simulink model "CarHalf_Vertical"  (R2018b)
settings: Solver=VariableStepAuto  StartTime=0.0  StopTime=10.0  RelTol=1e-3
values from neighbouring files (symbols this model uses):
  a = b    (= 1.4)    [CarQuarterParam.m]
  b = 1.4    [CarQuarterParam.m]
  Lamda = 1    [CarQuarterParam.m]
  speed = speedmph * 1000 * (1.609/3600)    (= 2.23472222222)    [CarQuarterParam.m]
settings Model: Creator=reece  LastModifiedBy=reece

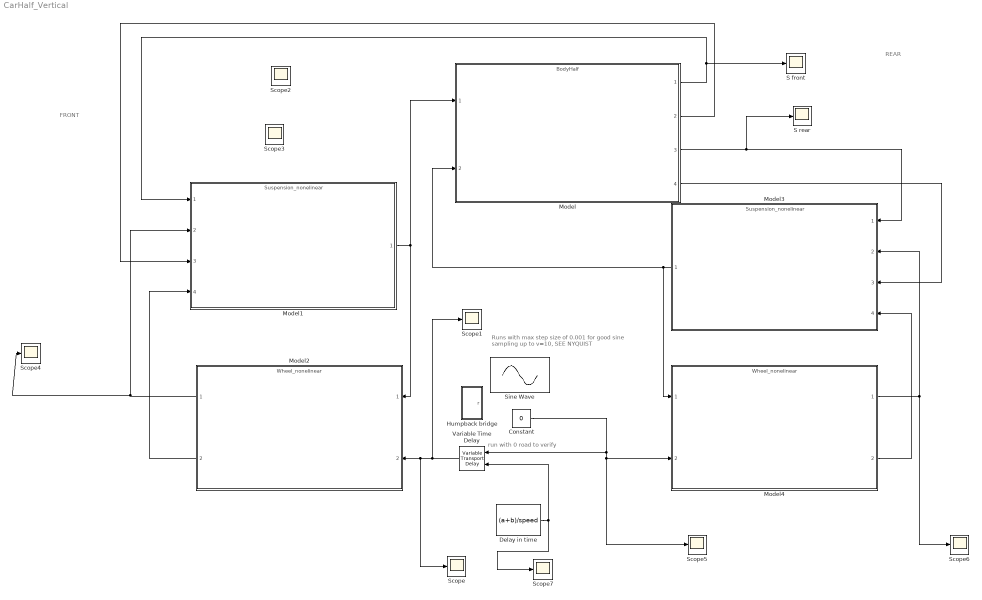
== system CarHalf_Vertical ==
  note: run with 0 road to verify
  note: Runs with max step size of 0.001 for good sine sampling up to v=10, SEE NYQUIST
  note: FRONT
  note: REAR
  Constant : Constant  Value=0
  Delay in time : Constant  Value=(a+b)/speed
  Humpback bridge : Subsystem  mask{h=2, L=20, v=speed}
      mask prompts: h "humpback height (m)"; L "humpback length (m)"; v "vehicle speed (m/s)"
  Model : ModelReference  ModelNameDialog=BodyHalf.slx  SimulationMode=Normal  ModelReferenceVersion=1.5
  Model1 : ModelReference  ModelNameDialog=Suspension_nonelinear.slx  SimulationMode=Normal  ModelReferenceVersion=1.10
  Model2 : ModelReference  ModelNameDialog=Wheel_nonelinear.slx  SimulationMode=Normal  ModelReferenceVersion=1.17
  Model3 : ModelReference  ModelNameDialog=Suspension_nonelinear.slx  SimulationMode=Normal  ModelReferenceVersion=1.10
  Model4 : ModelReference  ModelNameDialog=Wheel_nonelinear.slx  SimulationMode=Normal  ModelReferenceVersion=1.17
  S front : Scope
  S rear : Scope
  Scope{,1..7} (8 alike) : Scope
  Sine Wave : Sin  Frequency=(speed*2*pi)/Lamda  SampleTime=0
  Variable Time Delay : VariableTransportDelay  MaximumDelay=10
  wires:
  Constant/1 -> Variable Time Delay/1, Scope5/1, Model4/2
  Model1/1 -> Model/1, Model2/1
  Model4/1 -> Model3/2, Scope6/1
  Model/2 -> Model1/3
  Variable Time Delay/1 -> Scope1/1, Scope/1, Model2/2
  Model/3 -> S rear/1, Model3/1
  Model2/2 -> Model1/4
  Delay in time/1 -> Variable Time Delay/2, Scope7/1
  Model/1 -> S front/1, Model1/1
  Model/4 -> Model3/3
  Model4/2 -> Model3/4
  Model3/1 -> Model/2, Model4/1
  Model2/1 -> Scope4/1, Model1/2

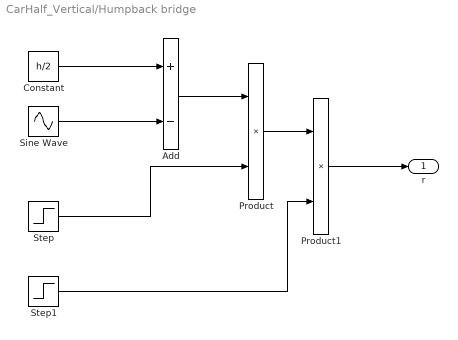
== system CarHalf_Vertical/Humpback bridge ==
  Add : Sum  Inputs=+-
  Constant : Constant  Value=h/2
  Product : Product
  Product1 : Product
  Sine Wave : Sin  Amplitude=h/2  Frequency=2*pi*v/L  Phase=pi/2  SampleTime=0
  Step : Step  Time=2*L/v  SampleTime=0
  Step1 : Step  Time=3*L/v  Before=1  After=0  SampleTime=0
  r : Outport
  wires:
  Constant/1 -> Add/1
  Sine Wave/1 -> Add/2
  Add/1 -> Product/1
  Step/1 -> Product/2
  Product/1 -> Product1/1
  Step1/1 -> Product1/2
  Product1/1 -> r/1
